simulink model "CL_Decoupled_Back"  (R2025a)
settings: Solver=ode113  StartTime=0.0  StopTime=1250  RelTol=1e-3
values from neighbouring files (symbols this model uses):
  h0 = [ 2, 2, 2, 2 ].'    [main_control.m]
  R1 = pidtune(Gs(1, 1), 'PI', 0.05)    [main_control.m]
  R2 = pidtune(Gs(2, 2), 'PI', 0.05)    [main_control.m]
  T12 = minreal(- Gs(1, 2) / Gs(1, 1))    [main_control.m]
  T21 = minreal(- Gs(2, 1) / Gs(2, 2))    [main_control.m]
  u_bar = [6.60003195923 9.28189672086]    [LQI_params.mat]    (also in linearize_4tanks.m = reshape(z_opt(5:6), [2, 1]))
  xv = 0:0.05:18    [main_control.m]
  ygamma1 = gamma1_fcn(xv)    [main_control.m]
  ygamma2 = gamma2_fcn(xv)    [main_control.m]
  yk1 = k1_fcn(xv)    [main_control.m]
  yk2 = k2_fcn(xv)    [main_control.m]
undefined symbols (not defined in the file or in its folder): AA
libraries: slpidlib x2, simulink x2, simulink_extras x2
settings Model: Creator=fabio  LastModifiedBy=oguzhanenes
settings OptimizationCC: BlockReduction=off  DefaultParameterBehavior=Inlined  BufferReuse=off  ReuseModelBlockBuffer=off
settings RTWCC: GPUComputeCapability=3.5

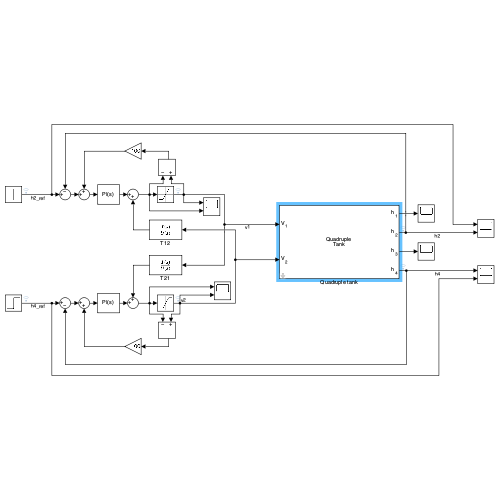
[thumbnail: Simulink's stored preview of the top-level diagram]
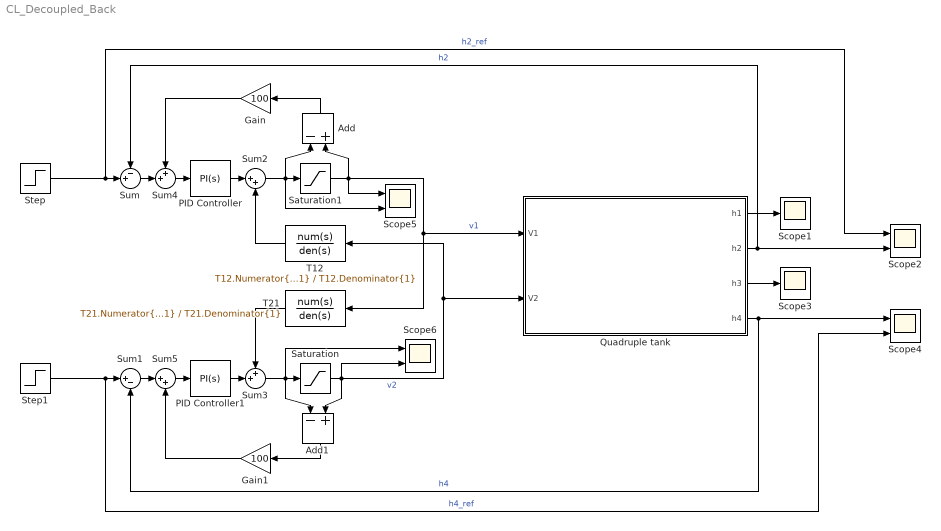
== system CL_Decoupled_Back ==
  Add : Sum  Inputs=-+
  Add1 : Sum  Inputs=-+
  Gain : Gain  Gain=100
  Gain1 : Gain  Gain=100
  PID Controller : slpidlib/PID Controller  Controller=PI  Form=Parallel  TimeDomain=Continuous-time  UseExternalTs=off  SampleTime=-1  IntegratorMethod=Forward Euler  FilterMethod=Forward Euler  ControllerParametersSource=internal  P=R1.Kp  I=R1.Ki  UseKiTs=off  D=0  UseExternalDerivativeSource=off  N=100  UseFilter=on  TunerSelectOption=Transfer Function Based (PID Tuner App)  InitialConditionSource=internal  InitialConditionForIntegrator=u_bar(1)  InitialConditionForFilter=0  DifferentiatorICPrevScaledInput=0  ExternalReset=none  TrackingMode=off  Kt=1  LimitOutput=off  SatLimitsSource=internal  UpperSaturationLimit=18  LowerSaturationLimit=0  LinearizeAsGain=on  AntiWindupMode=clamping  Kb=10  LimitIntegrator=off  UpperIntegratorSaturationLimit=inf  LowerIntegratorSaturationLimit=-inf  POutMin=[]  POutMax=[]  IOutMin=[]  IOutMax=[]  DOutMin=[]  DOutMax=[]  NOutMin=[]  NOutMax=[]  SumOutMin=[]  SumOutMax=[]  SaturationOutMin=[]  SaturationOutMax=[]  PParamMin=[]  PParamMax=[]  IParamMin=[]  IParamMax=[]  DParamMin=[]  DParamMax=[]  NParamMin=[]  NParamMax=[]  KbParamMin=[]  KbParamMax=[]  KtParamMin=[]  KtParamMax=[]  KbOutMin=[]  KbOutMax=[]  KtOutMin=[]  KtOutMax=[]  IntegratorOutMin=[]  IntegratorOutMax=[]  FilterOutMin=[]  FilterOutMax=[]  SumI1OutMin=[]  SumI1OutMax=[]  SumI2OutMin=[]  SumI2OutMax=[]  SumI3OutMin=[]  SumI3OutMax=[]  SumI4OutMin=[]  SumI4OutMax=[]  SumDOutMin=[]  SumDOutMax=[]  DifferentiatorOutMin=[]  DifferentiatorOutMax=[]  FilterDiffOutCoefMin=[]  FilterDiffOutCoefMax=[]  ReciprocalOutMin=[]  ReciprocalOutMax=[]  SumDenOutMin=[]  SumDenOutMax=[]  SumNumOutMin=[]  SumNumOutMax=[]  DivideOutMin=[]  DivideOutMax=[]  UdiffTsProdOutMin=[]  UdiffTsProdOutMax=[]  NTsProdOutMin=[]  NTsProdOutMax=[]  UintegralTsProdOutMin=[]  UintegralTsProdOutMax=[]  UngainTsProdOutMin=[]  UngainTsProdOutMax=[]  ClampingZeroOutDataTypeStr=Inherit: Inherit via back propagation  ClampingZeroOutMin=[]  ClampingZeroOutMax=[]  FilterDenConstantOutDataTypeStr=Inherit: Inherit via back propagation  FilterDenConstantOutMin=[]  FilterDenConstantOutMax=[]  PCopyOutDataTypeStr=Inherit: Inherit via back propagation  PCopyOutMin=[]  PCopyOutMax=[]  NCopyOutDataTypeStr=Inherit: Inherit via back propagation  NCopyOutMin=[]  NCopyOutMax=[]  IntegratorContinuousStateAttributes=''  IntegratorStateMustResolveToSignalObject=off  IntegratorRTWStateStorageClass=Auto  FilterContinuousStateAttributes=''  FilterStateMustResolveToSignalObject=off  FilterRTWStateStorageClass=Auto  ParallelPVariant=InternalParameters  IdealPVariant=Disabled  IVariant=InternalParameters  DVariant=Disabled  IntegratorVariant=Continuous  SatVariant=Disabled  AWVariant=Passthrough  PCopyVariant=Disabled  TRVariant=Disabled  FdbkBlocksVariant=Forward  IdealPFdbkVariant=Disabled  SatFdbkVariant=Disabled  DerivativeFilterVariant=Disabled  NVariant=Disabled  NCopyVariant=Disabled_SignalSpec  FilterICVariant=Disabled  IntegratorICVariant=InternalICs  ExternalResetVariant=Disabled  TRSumVariant=Passthrough  SumFdbkVariant=Disabled  SumVariant=Sum_PI  TsampFilterVariant=InternalTs  TsampNgainVariant=Passthrough  TsampIntegralVariant=Disabled_SignalSpec  ExternalSaturationOutDataTypeStr=Inherit: Same as second input  DerivativeSourceVariant=Disabled  PreIntVariant=InternalPreInt
  PID Controller1 : slpidlib/PID Controller  Controller=PI  Form=Parallel  TimeDomain=Continuous-time  UseExternalTs=off  SampleTime=-1  IntegratorMethod=Forward Euler  FilterMethod=Forward Euler  ControllerParametersSource=internal  P=R2.Kp  I=R2.Ki  UseKiTs=off  D=0  UseExternalDerivativeSource=off  N=100  UseFilter=on  TunerSelectOption=Transfer Function Based (PID Tuner App)  InitialConditionSource=internal  InitialConditionForIntegrator=u_bar(2)  InitialConditionForFilter=0  DifferentiatorICPrevScaledInput=0  ExternalReset=none  TrackingMode=off  Kt=1  LimitOutput=off  SatLimitsSource=internal  UpperSaturationLimit=18  LowerSaturationLimit=0  LinearizeAsGain=on  AntiWindupMode=clamping  Kb=10  LimitIntegrator=off  UpperIntegratorSaturationLimit=inf  LowerIntegratorSaturationLimit=-inf  POutMin=[]  POutMax=[]  IOutMin=[]  IOutMax=[]  DOutMin=[]  DOutMax=[]  NOutMin=[]  NOutMax=[]  SumOutMin=[]  SumOutMax=[]  SaturationOutMin=[]  SaturationOutMax=[]  PParamMin=[]  PParamMax=[]  IParamMin=[]  IParamMax=[]  DParamMin=[]  DParamMax=[]  NParamMin=[]  NParamMax=[]  KbParamMin=[]  KbParamMax=[]  KtParamMin=[]  KtParamMax=[]  KbOutMin=[]  KbOutMax=[]  KtOutMin=[]  KtOutMax=[]  IntegratorOutMin=[]  IntegratorOutMax=[]  FilterOutMin=[]  FilterOutMax=[]  SumI1OutMin=[]  SumI1OutMax=[]  SumI2OutMin=[]  SumI2OutMax=[]  SumI3OutMin=[]  SumI3OutMax=[]  SumI4OutMin=[]  SumI4OutMax=[]  SumDOutMin=[]  SumDOutMax=[]  DifferentiatorOutMin=[]  DifferentiatorOutMax=[]  FilterDiffOutCoefMin=[]  FilterDiffOutCoefMax=[]  ReciprocalOutMin=[]  ReciprocalOutMax=[]  SumDenOutMin=[]  SumDenOutMax=[]  SumNumOutMin=[]  SumNumOutMax=[]  DivideOutMin=[]  DivideOutMax=[]  UdiffTsProdOutMin=[]  UdiffTsProdOutMax=[]  NTsProdOutMin=[]  NTsProdOutMax=[]  UintegralTsProdOutMin=[]  UintegralTsProdOutMax=[]  UngainTsProdOutMin=[]  UngainTsProdOutMax=[]  ClampingZeroOutDataTypeStr=Inherit: Inherit via back propagation  ClampingZeroOutMin=[]  ClampingZeroOutMax=[]  FilterDenConstantOutDataTypeStr=Inherit: Inherit via back propagation  FilterDenConstantOutMin=[]  FilterDenConstantOutMax=[]  PCopyOutDataTypeStr=Inherit: Inherit via back propagation  PCopyOutMin=[]  PCopyOutMax=[]  NCopyOutDataTypeStr=Inherit: Inherit via back propagation  NCopyOutMin=[]  NCopyOutMax=[]  IntegratorContinuousStateAttributes=''  IntegratorStateMustResolveToSignalObject=off  IntegratorRTWStateStorageClass=Auto  FilterContinuousStateAttributes=''  FilterStateMustResolveToSignalObject=off  FilterRTWStateStorageClass=Auto  ParallelPVariant=InternalParameters  IdealPVariant=Disabled  IVariant=InternalParameters  DVariant=Disabled  IntegratorVariant=Continuous  SatVariant=Disabled  AWVariant=Passthrough  PCopyVariant=Disabled  TRVariant=Disabled  FdbkBlocksVariant=Forward  IdealPFdbkVariant=Disabled  SatFdbkVariant=Disabled  DerivativeFilterVariant=Disabled  NVariant=Disabled  NCopyVariant=Disabled_SignalSpec  FilterICVariant=Disabled  IntegratorICVariant=InternalICs  ExternalResetVariant=Disabled  TRSumVariant=Passthrough  SumFdbkVariant=Disabled  SumVariant=Sum_PI  TsampFilterVariant=InternalTs  TsampNgainVariant=Passthrough  TsampIntegralVariant=Disabled_SignalSpec  ExternalSaturationOutDataTypeStr=Inherit: Same as second input  DerivativeSourceVariant=Disabled  PreIntVariant=InternalPreInt
  Quadruple tank : Subsystem  mask{h_0=h0, A=AA, S=(4.44 / 2)^2 * pi * ones(1, 4), g=981}
      mask prompts: h_0 "Initial level"; A "Outlet section"; S "Tank section"; g "Gravity"
      mask DialogControl h_0 Tooltip: [cm]
      mask DialogControl A Tooltip: [cm^2]
      mask DialogControl S Tooltip: [cm^2]
      mask DialogControl g Tooltip: [cm/s^2]
      mask Display:
      | disp('Quadruple\nTank');
      | port_label('input', 1, 'V_1', 'interpreter', 'tex');
      | port_label('input', 2, 'V_2', 'interpreter', 'tex');
      | port_label('output', 1, 'h_1', 'interpreter', 'tex');
      | port_label('output', 2, 'h_2', 'interpreter', 'tex');
      | port_label('output', 3, 'h_3', 'interpreter', 'tex');
      | port_label('output', 4, 'h_4', 'interpreter', 'tex');
  Saturation : Saturate  UpperLimit=18  LowerLimit=0
  Saturation1 : Saturate  UpperLimit=18  LowerLimit=0
  Scope1 : Scope
      settings: ActiveDisplayYMinimum=-2.0625246465182427  ActiveDisplayYMaximum=26.178315574673771  DataLoggingVariableName=ScopeData4
  Scope{2,4..6} (4 alike) : Scope  NumInputPorts=2
      Scope2 settings: ActiveDisplayYMinimum=-1.5817016456473143  ActiveDisplayYMaximum=15.326560208481206
      Scope4 settings: ActiveDisplayYMinimum=-1.56954  ActiveDisplayYMaximum=15.46505  DataLoggingVariableName=ScopeData2
      Scope5 settings: ActiveDisplayYMinimum=5.9999103600366315  ActiveDisplayYMaximum=12.001126351956335
      Scope6 settings: ActiveDisplayYMinimum=5.2690587572817051  ActiveDisplayYMaximum=9.9881925769284479  DataLoggingVariableName=ScopeData5
  Scope3 : Scope
      settings: ActiveDisplayYMinimum=-1.992710088189084  ActiveDisplayYMaximum=24.600334799663312  DataLoggingVariableName=ScopeData3
  Step : Step  Time=500  Before=10  After=13  SampleTime=0
  Step1 : Step  Time=500  Before=10  After=10  SampleTime=0
  Sum : Sum  Inputs=-+|
  Sum1 : Sum  Inputs=|+-
  Sum2 : Sum  Inputs=|++
  Sum3 : Sum  Inputs=++|
  Sum4 : Sum  Inputs=++|
  Sum5 : Sum  Inputs=|++
  T12 : TransferFcn  Numerator=T12.Numerator{1}  Denominator=T12.Denominator{1}
  T21 : TransferFcn  Numerator=T21.Numerator{1}  Denominator=T21.Denominator{1}
  wires:
  PID Controller1/1 -> Sum3/2
  Step/1 -> Scope2/1, Sum/2  "h2_ref"
  Quadruple tank/2(h2) -> Scope2/2, Sum/1  "h2"
  Quadruple tank/1(h1) -> Scope1/1
  Quadruple tank/3(h3) -> Scope3/1
  Quadruple tank/4(h4) -> Scope4/1, Sum1/2  "h4"
  Step1/1 -> Scope4/2, Sum1/1  "h4_ref"
  PID Controller/1 -> Sum2/1
  T12/1 -> Sum2/2
  Sum2/1 -> Scope5/2, Add/1, Saturation1/1
  Sum3/1 -> Scope6/1, Add1/1, Saturation/1
  T21/1 -> Sum3/1
  Saturation/1 -> Scope6/2, T12/1, Quadruple tank/2(V2), Add1/2  "v2"
  Saturation1/1 -> T21/1, Quadruple tank/1(V1), Scope5/1, Add/2  "v1"
  Add/1 -> Gain/1
  Sum/1 -> Sum4/2
  Sum4/1 -> PID Controller/1
  Gain/1 -> Sum4/1
  Sum1/1 -> Sum5/1
  Sum5/1 -> PID Controller1/1
  Add1/1 -> Gain1/1
  Gain1/1 -> Sum5/2

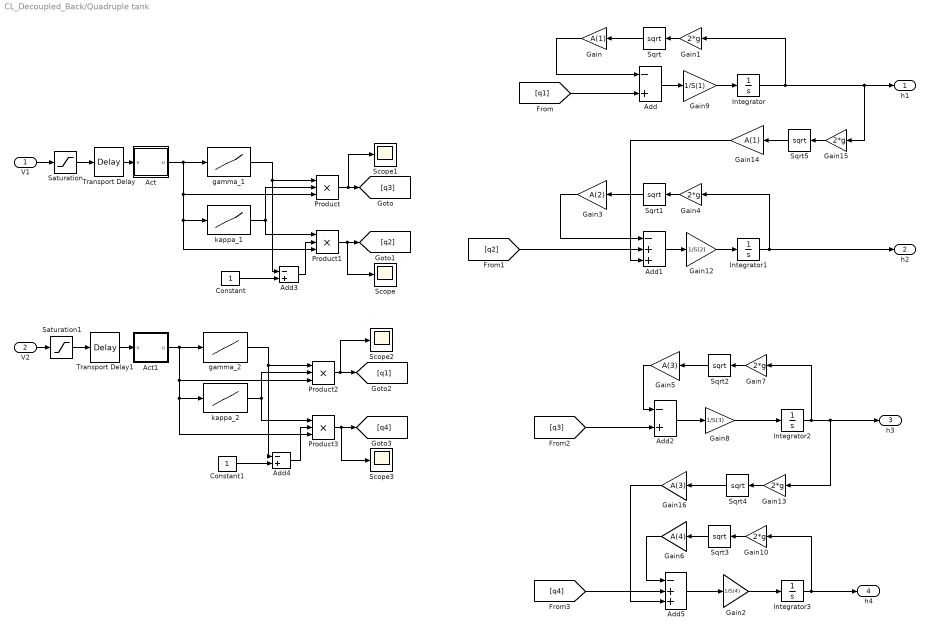
== system CL_Decoupled_Back/Quadruple tank ==
  V1 : Inport
  V2 : Inport  Port=2
  Act : Subsystem
  Act1 : Subsystem
  Add{,2..4} (4 alike) : Sum  Inputs=-+
  Add1 : Sum  Inputs=-++
  Add5 : Sum  Inputs=-++
  Constant : Constant
  Constant1 : Constant
  Gain : Gain  Gain=A(1)
  Gain{1,4,7,10,13,15} (6 alike) : Gain  Gain=2*g
  Gain12 : Gain  Gain=1/S(2)
  Gain14 : Gain  Gain=A(1)
  Gain16 : Gain  Gain=A(3)
  Gain2 : Gain  Gain=1/S(4)
  Gain3 : Gain  Gain=A(2)
  Gain5 : Gain  Gain=A(3)
  Gain6 : Gain  Gain=A(4)
  Gain8 : Gain  Gain=1/S(3)
  Gain9 : Gain  Gain=1/S(1)
  Integrator : Integrator  InitialCondition=h_0(1)  LimitOutput=on  UpperSaturationLimit=30  LowerSaturationLimit=0
  Integrator1 : Integrator  InitialCondition=h_0(2)  LimitOutput=on  UpperSaturationLimit=30  LowerSaturationLimit=0
  Integrator2 : Integrator  InitialCondition=h_0(3)  LimitOutput=on  UpperSaturationLimit=30  LowerSaturationLimit=0
  Integrator3 : Integrator  InitialCondition=h_0(4)  LimitOutput=on  UpperSaturationLimit=30  LowerSaturationLimit=0
  Product{,1..3} (4 alike) : Product  Inputs=3
  Saturation : Saturate  UpperLimit=18  LowerLimit=0
  Saturation1 : Saturate  UpperLimit=18  LowerLimit=0
  Scope{,1..3} (4 alike) : Scope
      Scope settings: ActiveDisplayYMinimum=-1  ActiveDisplayYMaximum=1  DataLoggingVariableName=ScopeData6
      Scope1 settings: ActiveDisplayYMinimum=-0.0309068585195216  ActiveDisplayYMaximum=0.11997221495064793  DataLoggingVariableName=ScopeData7
      Scope2 settings: ActiveDisplayYMinimum=-1.6797469057691881  ActiveDisplayYMaximum=15.117722151922697  DataLoggingVariableName=ScopeData8
      Scope3 settings: DataLoggingVariableName=ScopeData9
  Sqrt{,1..5} (6 alike) : Sqrt
  Transport Delay : TransportDelay  DelayTime=2
  Transport Delay1 : TransportDelay  DelayTime=2
  gamma_1 : Lookup_n-D  NumberOfTableDimensions=1  BreakpointsForDimension1=xv  Table=ygamma1  ExtrapMethod=Clip  UseLastTableValue=on  InternalRulePriority=Speed  RndMeth=Simplest
  gamma_2 : Lookup_n-D  NumberOfTableDimensions=1  BreakpointsForDimension1=xv  Table=ygamma2  ExtrapMethod=Clip  UseLastTableValue=on  InternalRulePriority=Speed  RndMeth=Simplest
  kappa_1 : Lookup_n-D  NumberOfTableDimensions=1  BreakpointsForDimension1=xv  Table=yk1  ExtrapMethod=Clip  UseLastTableValue=on  InternalRulePriority=Speed  RndMeth=Simplest
  kappa_2 : Lookup_n-D  NumberOfTableDimensions=1  BreakpointsForDimension1=xv  Table=yk2  ExtrapMethod=Clip  UseLastTableValue=on  InternalRulePriority=Speed  RndMeth=Simplest
  h1 : Outport
  h2 : Outport  Port=2
  h3 : Outport  Port=3
  h4 : Outport  Port=4
  wires:
  Integrator/1 -> Gain15/1, h1/1, Gain1/1
  Gain1/1 -> Sqrt/1
  Sqrt/1 -> Gain/1
  Gain/1 -> Add/1
  [q1] -> Add/2
  Add1/1 -> Gain12/1
  Integrator1/1 -> Gain4/1, h2/1
  Gain4/1 -> Sqrt1/1
  Add2/1 -> Gain8/1
  Gain7/1 -> Sqrt2/1
  Sqrt2/1 -> Gain5/1
  Gain6/1 -> Add5/1
  Sqrt3/1 -> Gain6/1
  Gain10/1 -> Sqrt3/1
  Integrator3/1 -> Gain10/1, h4/1
  [q4] -> Add5/2
  Sqrt4/1 -> Gain16/1
  Gain13/1 -> Sqrt4/1
  Integrator2/1 -> Gain7/1, h3/1, Gain13/1
  Sqrt1/1 -> Gain3/1
  Gain3/1 -> Add1/1
  Gain5/1 -> Add2/1
  Gain15/1 -> Sqrt5/1
  Sqrt5/1 -> Gain14/1
  Gain14/1 -> Add1/3
  [q2] -> Add1/2
  [q3] -> Add2/2
  Gain16/1 -> Add5/3
  gamma_1/1 -> Add3/1, Product/1
  Constant/1 -> Add3/2
  kappa_1/1 -> Product/2, Product1/1
  Add3/1 -> Product1/2
  Product/1 -> Scope1/1, [q3]
  Product1/1 -> Scope/1, [q2]
  kappa_2/1 -> Product3/1, Product2/2
  Product2/1 -> Scope2/1, [q1]
  Constant1/1 -> Add4/2
  gamma_2/1 -> Add4/1, Product2/1
  Product3/1 -> Scope3/1, [q4]
  Add4/1 -> Product3/2
  Gain12/1 -> Integrator1/1
  Add/1 -> Gain9/1
  Gain9/1 -> Integrator/1
  Gain8/1 -> Integrator2/1
  Add5/1 -> Gain2/1
  Gain2/1 -> Integrator3/1
  Act/1(u) -> gamma_1/1, Product/3, kappa_1/1, Product1/3
  Act1/1(u) -> gamma_2/1, Product2/3, kappa_2/1, Product3/3
  Transport Delay/1 -> Act/1(v)
  V1/1 -> Saturation/1
  Saturation/1 -> Transport Delay/1
  Saturation1/1 -> Transport Delay1/1
  V2/1 -> Saturation1/1
  Transport Delay1/1 -> Act1/1(v)

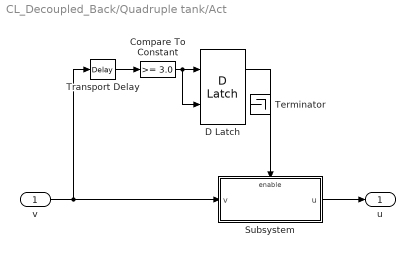
== system CL_Decoupled_Back/Quadruple tank/Act ==
  v : Inport
  Compare To Constant : simulink/Logic and Bit Operations/Compare To Constant  relop=>=  const=3.0  OutDataTypeStr=boolean
  D Latch : simulink_extras/Flip Flops/D Latch
  Subsystem : Subsystem
  Terminator : Terminator
  Transport Delay : TransportDelay  DelayTime=4
  u : Outport
  wires:
  v/1 -> Transport Delay/1, Subsystem/1(v)
  D Latch/1 -> Subsystem/Enable
  Subsystem/1(u) -> u/1
  Transport Delay/1 -> Compare To Constant/1
  Compare To Constant/1 -> D Latch/2, D Latch/1

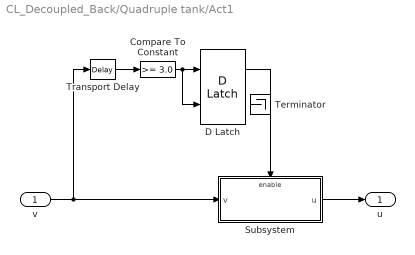
== system CL_Decoupled_Back/Quadruple tank/Act1 ==
  v : Inport
  Compare To Constant : simulink/Logic and Bit Operations/Compare To Constant  relop=>=  const=3.0  OutDataTypeStr=boolean
  D Latch : simulink_extras/Flip Flops/D Latch
  Subsystem : Subsystem
  Terminator : Terminator
  Transport Delay : TransportDelay  DelayTime=4
  u : Outport
  wires:
  v/1 -> Transport Delay/1, Subsystem/1(v)
  D Latch/1 -> Subsystem/Enable
  Subsystem/1(u) -> u/1
  Transport Delay/1 -> Compare To Constant/1
  Compare To Constant/1 -> D Latch/2, D Latch/1

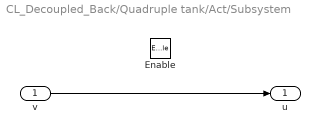
== system CL_Decoupled_Back/Quadruple tank/Act/Subsystem ==
  v : Inport
  Enable : EnablePort
  u : Outport
  wires:
  v/1 -> u/1

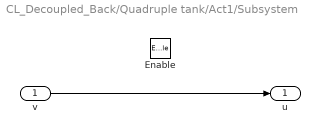
== system CL_Decoupled_Back/Quadruple tank/Act1/Subsystem ==
  v : Inport
  Enable : EnablePort
  u : Outport
  wires:
  v/1 -> u/1
